simulink model "GFLIB_VMin_BAM_F32"  (Simulink 8.3)
settings: Solver=ode45  StartTime=0.0  StopTime=10.0  RelTol=1e-3
undefined symbols (not defined in the file): N
settings Model: Creator=B37097  LastModifiedBy=nxa18952
settings DataIOCC: SignalLoggingSaveFormat=Dataset
settings DebuggingCC: UnderspecifiedInitializationDetection=Simplified  StateNameClashWarn=none
settings GRTTargetCC: CombineOutputUpdateFcns=on  GRTInterface=off

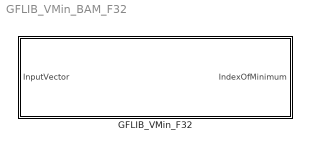
== system GFLIB_VMin_BAM_F32 ==
  GFLIB_VMin_F32 : Subsystem  mask(GFLIB_VMin_F32){N=N}
      mask prompts: N "Vector length"
      mask help: Bit accurate model of GFLIB_VMin function, which finds the index of a vector minimum.
      mask init:
      | pos = get_param(gcb, 'Position');width = pos(3) - pos(1); height = pos(4) - pos(2);tX=width/2;tY=height*0.9;
      mask Display: color('black');port_label('input',1,'InputVector');port_label('output',1,'IndexOfMinimum');color('black');disp('GFLIB_VMin_F32');color('blue');text(tX,tY, 'BAM', 'horizontalAlignment', 'center');

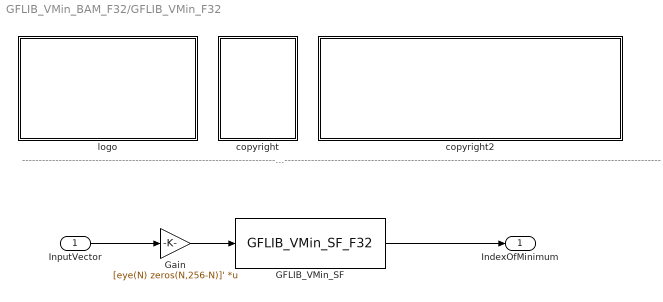
== system GFLIB_VMin_BAM_F32/GFLIB_VMin_F32 ==
  note: ---------------------------------------------------------------------------------------------------------------------------------------------------------------------------------------------------
  InputVector : Inport
  GFLIB_VMin_SF : S-Function  FunctionName=GFLIB_VMin_SF_F32  Parameters=N  EnableBusSupport=off
  Gain : Gain  Gain=[eye(N) zeros(N,256-N)]'  Multiplication=Matrix(K*u)  OutDataTypeStr=int32
  copyright : Subsystem
      mask Display: text(10,90,'FILE:');text(10,75,'DESRIPTION:');text(10,60,'COPYRIGHT:');text(10,45,'VERSION:');text(10,30,'DATE:')
  copyright2 : Subsystem
      mask Display: text(10,90,'GFLIB_VMin_BAM_F32.mdl');text(10,75,'Vector minimum');text(10,60,'NXP');text(10,45,'1.0');text(10,30,'18-Jan-2018');
  logo : Subsystem
      mask Display: image(imread('logo.jpg'))
  IndexOfMinimum : Outport
  wires:
  InputVector/1 -> Gain/1
  Gain/1 -> GFLIB_VMin_SF/1
  GFLIB_VMin_SF/1 -> IndexOfMinimum/1

== system GFLIB_VMin_BAM_F32/GFLIB_VMin_F32/copyright ==

== system GFLIB_VMin_BAM_F32/GFLIB_VMin_F32/copyright2 ==

== system GFLIB_VMin_BAM_F32/GFLIB_VMin_F32/logo ==
